simulink model "Sample594"  (R2021b)
settings: Solver=VariableStepAuto  StartTime=0.0  StopTime=10.0  RelTol=1e-3
undefined symbols (not defined in the file): DiscIntNeverNeededParam, magnitude, Newton, Raphson
libraries: simulink x402, pid_lib x98
(part 2 of 14)

== system Sample594/cfblk7/cfblk9 ==
  cfblk1 : Inport
  cfblk10 : Delay  SampleTime=1
  cfblk11 : Delay  SampleTime=1
  cfblk3 : simulink/Discrete/Difference  ICPrevInput=0.0  OutMin=[]  OutMax=[]  OutDataTypeStr=Inherit: Inherit via back propagation  OutDataType=fixdt(1, 16)  OutScaling=2^-10  DoSatur=off
  cfblk4 : simulink/Math Operations/Slider Gain  gain=1  low=0  high=2
  cfblk5 : Sum  Inputs=+
  cfblk6 : Subsystem
  cfblk7 : Subsystem
  cfblk8 : Subsystem
  cfblk9 : Delay  SampleTime=1
  cfblk2 : Outport
  wires:
  cfblk3/1 -> cfblk5/1
  cfblk1/1 -> cfblk2/1, cfblk6/2(cfblk15)
  cfblk8/1(cfblk2) -> cfblk9/1, cfblk10/1
  cfblk7/1(cfblk2) -> cfblk8/1(cfblk1)
  cfblk5/1 -> cfblk7/1(cfblk1), cfblk11/1
  cfblk4/1 -> cfblk7/2(cfblk7), cfblk7/3(cfblk8), cfblk7/4(cfblk9), cfblk3/1
  cfblk6/1(cfblk2) -> cfblk4/1
  cfblk9/1 -> cfblk6/1(cfblk1)
  cfblk10/1 -> cfblk6/3(cfblk16)
  cfblk11/1 -> cfblk6/4(cfblk17)

== system Sample594/cfblk8/cfblk10 ==
  cfblk1 : Inport
  cfblk9 : Inport  Port=2
  cfblk3 : Delay  DelayLengthSource=Input port  SampleTime=1
      settings: InputPortMap=u0,p1
  cfblk4 : Polyval  Coefs=[ +2.081618890e-019, -1.441693666e-014, +4.719686976e-010, -8.536869453e-006, +1.621573104e-001, -8.087801117e+001 ]
  cfblk5 : Assignment  DiagnosticForDimensions=Warning  IndexOptions=Index vector (dialog)  Indices=1  OutputSizes=1
  cfblk6 : Polyval  Coefs=[ +2.081618890e-019, -1.441693666e-014, +4.719686976e-010, -8.536869453e-006, +1.621573104e-001, -8.087801117e+001 ]
  cfblk7 : Constant  Value=[-685362202.844304]  SampleTime=1
  cfblk8 : Subsystem
  cfblk2 : Outport
  cfblk10 : Outport  Port=2
  cfblk11 : Outport  Port=3
  wires:
  cfblk5/1 -> cfblk6/1
  cfblk6/1 -> cfblk4/1
  cfblk8/1(cfblk2) -> cfblk2/1
  cfblk8/2(cfblk15) -> cfblk11/1
  cfblk1/1 -> cfblk5/1, cfblk8/4(cfblk14)
  cfblk9/1 -> cfblk5/2, cfblk8/3(cfblk13)
  cfblk4/1 -> cfblk10/1
  cfblk7/1 -> cfblk3/1, cfblk3/2
  cfblk3/1 -> cfblk8/1(cfblk1), cfblk8/2(cfblk12)

== system Sample594/cfblk8/cfblk11 ==
  cfblk1 : Inport
  cfblk13 : Inport  Port=2
  cfblk14 : Inport  Port=3
  cfblk10 : Subsystem
  cfblk11 : Subsystem
  cfblk12 : Subsystem
  cfblk15 : Delay  SampleTime=1
  cfblk16 : Delay  SampleTime=1
  cfblk3 : simulink/Discrete/Tapped Delay  vinit=0.0  samptime=-1  NumDelays=1  DelayOrder=Oldest  includeCurrent=off
  cfblk4 : DiscreteFilter  SampleTime=1
  cfblk5 : Abs
  cfblk6 : Reshape
  cfblk7 : simulink/Math Operations/Slider Gain  gain=1  low=0  high=2
  cfblk8 : PermuteDimensions
  cfblk9 : Subsystem
  cfblk2 : Outport
  wires:
  cfblk12/1(cfblk2) -> cfblk8/1
  cfblk13/1 -> cfblk6/1
  cfblk8/1 -> cfblk7/1
  cfblk7/1 -> cfblk4/1
  cfblk1/1 -> cfblk12/1(cfblk1)
  cfblk6/1 -> cfblk10/1(cfblk1)
  cfblk10/1(cfblk2) -> cfblk5/1
  cfblk4/1 -> cfblk9/1(cfblk1)
  cfblk14/1 -> cfblk11/1(cfblk1)
  cfblk9/2(cfblk7) -> cfblk11/2(cfblk13)
  cfblk12/2(cfblk16) -> cfblk9/2(cfblk6)
  cfblk10/2(cfblk12) -> cfblk11/3(cfblk14)
  cfblk9/3(cfblk8) -> cfblk2/1
  cfblk3/1 -> cfblk10/2(cfblk11)
  cfblk9/1(cfblk2) -> cfblk15/1
  cfblk15/1 -> cfblk12/2(cfblk15)
  cfblk5/1 -> cfblk16/1
  cfblk16/1 -> cfblk3/1

== system Sample594/cfblk8/cfblk12 ==
  cfblk1 : Inport
  cfblk13 : Inport  Port=2
  cfblk10 : Subsystem
  cfblk11 : Subsystem
  cfblk12 : If  IfExpression=u1 >= 0  SampleTime=1
  cfblk15 : Subsystem  TreatAsAtomicUnit=on
  cfblk16 : Subsystem  TreatAsAtomicUnit=on
  cfblk17 : Delay  SampleTime=1
  cfblk18 : Delay  SampleTime=1
  cfblk3 : Delay  ShowEnablePort=on  SampleTime=1
      settings: InputPortMap=u0,e6
  cfblk4 : pid_lib/PID Controller  Controller=PID  Form=Parallel  TimeDomain=Discrete-time  UseExternalTs=off  SampleTime=1  IntegratorMethod=Forward Euler  FilterMethod=Forward Euler  ControllerParametersSource=internal  P=1  I=1  D=0  UseFilter=on  N=100  TunerSelectOption=Transfer Function Based (PID Tuner App)  InitialConditionSource=internal  InitialConditionForIntegrator=0  InitialConditionForFilter=0  DifferentiatorICPrevScaledInput=0  ExternalReset=none  TrackingMode=off  Kt=1  LimitOutput=off  SatLimitsSource=internal  UpperSaturationLimit=inf  LowerSaturationLimit=-inf  LinearizeAsGain=off  AntiWindupMode=none  Kb=1  POutMin=[]  POutMax=[]  IOutMin=[]  IOutMax=[]  DOutMin=[]  DOutMax=[]  NOutMin=[]  NOutMax=[]  SumOutMin=[]  SumOutMax=[]  SaturationOutMin=[]  SaturationOutMax=[]  PParamMin=[]  PParamMax=[]  IParamMin=[]  IParamMax=[]  DParamMin=[]  DParamMax=[]  NParamMin=[]  NParamMax=[]  KbParamMin=[]  KbParamMax=[]  KtParamMin=[]  KtParamMax=[]  KbOutMin=[]  KbOutMax=[]  KtOutMin=[]  KtOutMax=[]  IntegratorOutMin=[]  IntegratorOutMax=[]  FilterOutMin=[]  FilterOutMax=[]  SumI1OutMin=[]  SumI1OutMax=[]  SumI2OutMin=[]  SumI2OutMax=[]  SumI3OutMin=[]  SumI3OutMax=[]  SumI4OutMin=[]  SumI4OutMax=[]  SumDOutMin=[]  SumDOutMax=[]  DifferentiatorOutMin=[]  DifferentiatorOutMax=[]  FilterDiffOutCoefMin=[]  FilterDiffOutCoefMax=[]  ReciprocalOutMin=[]  ReciprocalOutMax=[]  SumDenOutMin=[]  SumDenOutMax=[]  SumNumOutMin=[]  SumNumOutMax=[]  DivideOutMin=[]  DivideOutMax=[]  UdiffTsProdOutMin=[]  UdiffTsProdOutMax=[]  NTsProdOutMin=[]  NTsProdOutMax=[]  UintegralTsProdOutMin=[]  UintegralTsProdOutMax=[]  UngainTsProdOutMin=[]  UngainTsProdOutMax=[]  IntegratorContinuousStateAttributes=''  IntegratorStateMustResolveToSignalObject=off  IntegratorRTWStateStorageClass=Auto  FilterContinuousStateAttributes=''  FilterStateMustResolveToSignalObject=off  FilterRTWStateStorageClass=Auto  ParallelPVariant=InternalParameters  IdealPVariant=Disabled  IVariant=InternalParameters  DVariant=InternalParameters  IntegratorVariant=Discrete  SatVariant=Disabled  AWVariant=Passthrough  PCopyVariant=Disabled  TRVariant=Disabled  FdbkBlocksVariant=Forward  IdealPFdbkVariant=Disabled  SatFdbkVariant=Disabled  DerivativeFilterVariant=ForwardEulerFilter  NVariant=InternalParameters  NCopyVariant=Disabled  FilterICVariant=InternalICsFilter  IntegratorICVariant=InternalICs  ExternalResetVariant=Disabled  TRSumVariant=Passthrough  SumFdbkVariant=Disabled  SumVariant=Sum_PID  TsampFilterVariant=InternalTs  TsampNgainVariant=Passthrough  TsampIntegralVariant=Passthrough  ExternalSaturationOutDataTypeStr=Inherit: Same as second input
  cfblk5 : Rounding
  cfblk6 : PermuteDimensions
  cfblk7 : Polyval  Coefs=[ +2.081618890e-019, -1.441693666e-014, +4.719686976e-010, -8.536869453e-006, +1.621573104e-001, -8.087801117e+001 ]
  cfblk8 : Constant  Value=[-411590028.519686]  SampleTime=1
  cfblk9 : Subsystem
  cfblk2 : Outport
  cfblk14 : Outport  Port=2
  wires:
  cfblk11/1(cfblk2) -> cfblk4/1
  cfblk8/1 -> cfblk11/1(cfblk1)
  cfblk13/1 -> cfblk6/1
  cfblk4/1 -> cfblk3/1
  cfblk6/1 -> cfblk10/1(cfblk1)
  cfblk10/1(cfblk2) -> cfblk9/1(cfblk1)
  cfblk7/1 -> cfblk16/2(cfblk16)
  cfblk9/1(cfblk2) -> cfblk2/1
  cfblk5/1 -> cfblk7/1
  cfblk16/1(cfblk2) -> cfblk15/1(cfblk1)
  cfblk1/1 -> cfblk5/1, cfblk3/2
  cfblk3/1 -> cfblk14/1
  cfblk9/2(cfblk11) -> cfblk15/2(cfblk16)
  cfblk9/3(cfblk12) -> cfblk12/1
  cfblk12/1 -> cfblk15/Action
  cfblk12/2 -> cfblk16/Action
  cfblk15/1(cfblk2) -> cfblk17/1
  cfblk17/1 -> cfblk16/1(cfblk1)
  cfblk15/2(cfblk17) -> cfblk18/1
  cfblk18/1 -> cfblk16/3(cfblk17)

== system Sample594/cfblk8/cfblk13 ==
  cfblk1 : Inport
  cfblk6 : Inport  Port=2
  cfblk7 : Inport  Port=3
  cfblk3 : Gain  Gain=[833103995.126030]
  cfblk4 : Constant  Value=[-958629368.502449]  SampleTime=1
  cfblk5 : Subsystem
  cfblk2 : Outport
  wires:
  cfblk6/1 -> cfblk3/1
  cfblk5/1(cfblk2) -> cfblk2/1
  cfblk1/1 -> cfblk5/1(cfblk1)
  cfblk7/1 -> cfblk5/2(cfblk8)

== system Sample594/cfblk8/cfblk9 ==
  cfblk1 : Inport
  cfblk11 : Inport  Port=2
  cfblk12 : Inport  Port=3
  cfblk10 : Subsystem
  cfblk13 : Delay  SampleTime=1
  cfblk3 : simulink/Math Operations/MinMax Running Resettable  Function=min  vinit=0.0
  cfblk4 : Rounding
  cfblk5 : UnaryMinus
  cfblk6 : Subsystem
  cfblk7 : Subsystem
  cfblk8 : Subsystem
  cfblk9 : Subsystem
  cfblk2 : Outport
  wires:
  cfblk1/1 -> cfblk4/1, cfblk6/5(cfblk11)
  cfblk10/1(cfblk2) -> cfblk7/1(cfblk1)
  cfblk8/1(cfblk2) -> cfblk10/1(cfblk1)
  cfblk8/2(cfblk8) -> cfblk5/1
  cfblk5/1 -> cfblk9/1(cfblk1)
  cfblk12/1 -> cfblk3/1, cfblk6/3(cfblk9)
  cfblk7/1(cfblk2) -> cfblk6/1(cfblk1)
  cfblk6/1(cfblk2) -> cfblk2/1, cfblk13/1
  cfblk3/1 -> cfblk8/1(cfblk1)
  cfblk4/1 -> cfblk8/2(cfblk7), cfblk6/4(cfblk10)
  cfblk9/1(cfblk2) -> cfblk6/2(cfblk8), cfblk7/3(cfblk10)
  cfblk11/1 -> cfblk3/2
  cfblk13/1 -> cfblk7/2(cfblk9)

== system Sample594/cfblk9/cfblk14 ==
  cfblk1 : Inport
  cfblk10 : Inport  Port=2
  cfblk11 : Inport  Port=3
  cfblk12 : Inport  Port=4
  cfblk13 : Inport  Port=5
  cfblk17 : Delay  SampleTime=1
  cfblk3 : DiscreteZeroPole  Poles=[0 0.5]  Gain=1
  cfblk4 : DiscreteZeroPole  Poles=[0 0.5]  Gain=1
  cfblk5 : Sum  Inputs=+-
  cfblk6 : DotProduct  InputSameDT=on  OutDataTypeStr=Inherit: Inherit via internal rule
  cfblk7 : Constant  Value=[-386291814.551287]  SampleTime=1
  cfblk8 : Subsystem
  cfblk9 : Subsystem
  cfblk2 : Outport
  cfblk14 : Outport  Port=2
  cfblk15 : Outport  Port=3
  cfblk16 : Outport  Port=4
  wires:
  cfblk10/1 -> cfblk8/1(cfblk1)
  cfblk1/1 -> cfblk15/1, cfblk8/3(cfblk8)
  cfblk5/1 -> cfblk14/1
  cfblk8/1(cfblk2) -> cfblk9/1(cfblk1)
  cfblk12/1 -> cfblk5/1
  cfblk6/1 -> cfblk16/1
  cfblk11/1 -> cfblk4/1
  cfblk9/1(cfblk2) -> cfblk3/1
  cfblk7/1 -> cfblk5/2
  cfblk13/1 -> cfblk6/1
  cfblk4/1 -> cfblk6/2, cfblk2/1, cfblk9/2(cfblk12)
  cfblk3/1 -> cfblk17/1
  cfblk17/1 -> cfblk8/2(cfblk7)

== system Sample594/cfblk11/cfblk10/cfblk10 ==
  cfblk1 : Inport
  cfblk10 : Subsystem
  cfblk{11..14} (4 alike) : Delay
  cfblk3 : Abs
  cfblk4 : Sum  Inputs=--
  cfblk5 : simulink/Math Operations/Slider Gain  gain=1  low=0  high=2
  cfblk6 : Signum
  cfblk7 : Subsystem
  cfblk8 : Subsystem
  cfblk9 : Subsystem
  cfblk2 : Outport
  wires:
  cfblk3/1 -> cfblk7/3(cfblk15), cfblk14/1
  cfblk4/1 -> cfblk10/1(cfblk1), cfblk7/4(cfblk16)
  cfblk5/1 -> cfblk4/2
  cfblk8/1(cfblk2) -> cfblk2/1
  cfblk8/2(cfblk10) -> cfblk6/1
  cfblk10/1(cfblk2) -> cfblk3/1, cfblk13/1
  cfblk1/1 -> cfblk8/3(cfblk9), cfblk7/2(cfblk14)
  cfblk8/3(cfblk11) -> cfblk9/2(cfblk9)
  cfblk9/1(cfblk2) -> cfblk7/1(cfblk1), cfblk5/1, cfblk7/5(cfblk17)
  cfblk6/1 -> cfblk11/1
  cfblk11/1 -> cfblk8/1(cfblk1)
  cfblk7/1(cfblk2) -> cfblk12/1
  cfblk12/1 -> cfblk8/2(cfblk8)
  cfblk13/1 -> cfblk9/1(cfblk1)
  cfblk14/1 -> cfblk4/1

== system Sample594/cfblk11/cfblk10/cfblk11 ==
  cfblk1 : Inport
  cfblk10 : Inport  Port=2
  cfblk11 : Delay
  cfblk12 : Delay
  cfblk13 : Delay
  cfblk3 : DiscreteIntegrator  SampleTime=-1  ICPrevOutput=DiscIntNeverNeededParam  ICPrevScaledInput=DiscIntNeverNeededParam
  cfblk4 : simulink/Math Operations/Slider Gain  gain=1  low=0  high=2
  cfblk5 : Abs
  cfblk6 : Sqrt  SaturateOnIntegerOverflow=on
  cfblk7 : Subsystem
  cfblk8 : Subsystem
  cfblk9 : Subsystem
  cfblk2 : Outport
  wires:
  cfblk8/1(cfblk2) -> cfblk6/1
  cfblk1/1 -> cfblk5/1
  cfblk7/1(cfblk2) -> cfblk4/1
  cfblk9/1(cfblk2) -> cfblk3/1
  cfblk6/1 -> cfblk7/2(cfblk14), cfblk9/3(cfblk14)
  cfblk10/1 -> cfblk8/2(cfblk13)
  cfblk8/2(cfblk15) -> cfblk7/3(cfblk15)
  cfblk8/3(cfblk16) -> cfblk2/1
  cfblk5/1 -> cfblk9/2(cfblk13), cfblk8/3(cfblk14)
  cfblk3/1 -> cfblk11/1
  cfblk11/1 -> cfblk9/1(cfblk1)
  cfblk4/1 -> cfblk12/1
  cfblk12/1 -> cfblk7/1(cfblk1)
  cfblk7/2(cfblk16) -> cfblk13/1
  cfblk13/1 -> cfblk8/1(cfblk1)

== system Sample594/cfblk11/cfblk10/cfblk12 ==
  cfblk1 : Inport
  cfblk10 : Inport  Port=2
  cfblk11 : Inport  Port=3
  cfblk3 : DiscreteTransferFcn
  cfblk4 : Sqrt  Operator=rSqrt  AlgorithmType=Newton-Raphson  SaturateOnIntegerOverflow=on
  cfblk5 : simulink/Math Operations/MinMax Running Resettable  Function=min  vinit=0.0
  cfblk6 : Sum  Inputs=--
  cfblk7 : Sin  TimeSource=Use external signal  SampleTime=0
  cfblk8 : Sqrt  Operator=rSqrt  AlgorithmType=Newton-Raphson  SaturateOnIntegerOverflow=on
  cfblk9 : Subsystem
  cfblk2 : Outport
  wires:
  cfblk11/1 -> cfblk8/1, cfblk9/6(cfblk14)
  cfblk8/1 -> cfblk3/1, cfblk9/3(cfblk11), cfblk9/5(cfblk13), cfblk9/7(cfblk15)
  cfblk7/1 -> cfblk2/1, cfblk9/1(cfblk1)
  cfblk4/1 -> cfblk6/1
  cfblk1/1 -> cfblk6/2
  cfblk3/1 -> cfblk4/1, cfblk9/4(cfblk12)
  cfblk5/1 -> cfblk7/1
  cfblk6/1 -> cfblk5/1
  cfblk10/1 -> cfblk5/2, cfblk9/2(cfblk10)

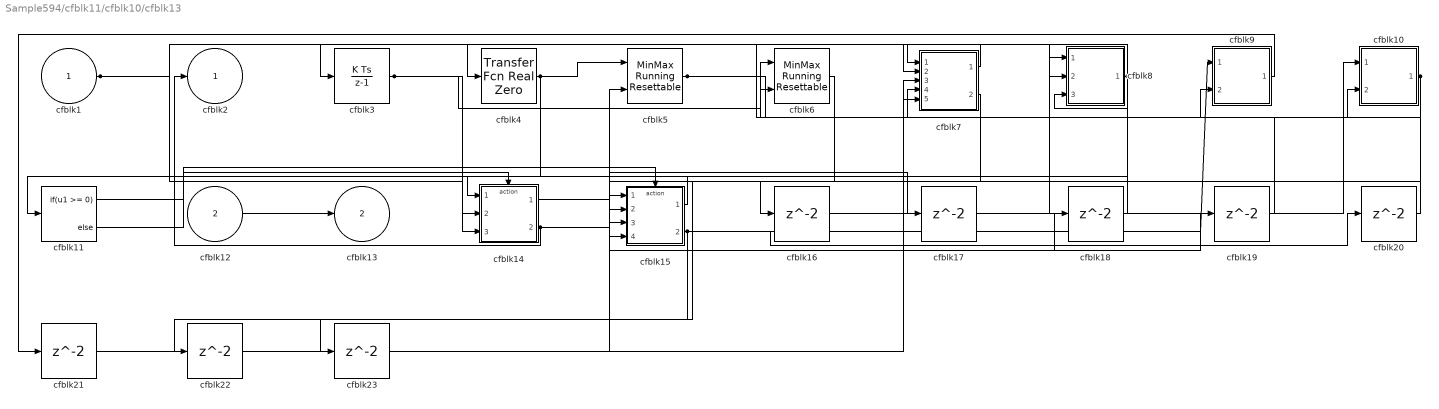
== system Sample594/cfblk11/cfblk10/cfblk13 ==
  cfblk1 : Inport
  cfblk12 : Inport  Port=2
  cfblk10 : Subsystem
  cfblk11 : If  IfExpression=u1 >= 0  SampleTime=1
  cfblk14 : Subsystem  TreatAsAtomicUnit=on
  cfblk15 : Subsystem  TreatAsAtomicUnit=on
  cfblk{16..23} (8 alike) : Delay
  cfblk3 : DiscreteIntegrator  SampleTime=-1  ICPrevOutput=DiscIntNeverNeededParam  ICPrevScaledInput=DiscIntNeverNeededParam
  cfblk4 : simulink/Discrete/Transfer Fcn Real Zero  ZeroZ=0.75  ICPrevInput=0.0  DoSatur=off
      settings: SourceProductBaseCode=SL
  cfblk5 : simulink/Math Operations/MinMax Running Resettable  Function=min  vinit=0.0
  cfblk6 : simulink/Math Operations/MinMax Running Resettable  Function=min  vinit=0.0
  cfblk7 : Subsystem
  cfblk8 : Subsystem
  cfblk9 : Subsystem
  cfblk2 : Outport
  cfblk13 : Outport  Port=2
  wires:
  cfblk8/1(cfblk2) -> cfblk4/1, cfblk11/1, cfblk7/2(cfblk13), cfblk15/3(cfblk13)
  cfblk14/2(cfblk17) -> cfblk2/1, cfblk18/1, cfblk19/1
  cfblk3/1 -> cfblk6/1, cfblk15/4(cfblk14)
  cfblk10/1(cfblk2) -> cfblk7/4(cfblk15), cfblk16/1
  cfblk15/1(cfblk2) -> cfblk14/1(cfblk1)
  cfblk4/1 -> cfblk5/1, cfblk14/3(cfblk16)
  cfblk1/1 -> cfblk8/2(cfblk9), cfblk14/2(cfblk15)
  cfblk7/1(cfblk2) -> cfblk3/1
  cfblk6/1 -> cfblk15/2(cfblk12)
  cfblk12/1 -> cfblk13/1
  cfblk5/1 -> cfblk10/2(cfblk7), cfblk7/1(cfblk1), cfblk9/2(cfblk11)
  cfblk15/2(cfblk15) -> cfblk9/1(cfblk1), cfblk20/1, cfblk22/1
  cfblk11/1 -> cfblk14/Action
  cfblk11/2 -> cfblk15/Action
  cfblk16/1 -> cfblk8/1(cfblk1)
  cfblk14/1(cfblk2) -> cfblk17/1
  cfblk17/1 -> cfblk10/1(cfblk1)
  cfblk18/1 -> cfblk8/3(cfblk10)
  cfblk19/1 -> cfblk7/3(cfblk14)
  cfblk20/1 -> cfblk6/2
  cfblk9/1(cfblk2) -> cfblk21/1
  cfblk21/1 -> cfblk15/1(cfblk1)
  cfblk22/1 -> cfblk7/5(cfblk16)
  cfblk7/2(cfblk17) -> cfblk23/1
  cfblk23/1 -> cfblk5/2

== system Sample594/cfblk11/cfblk11/cfblk10 ==
  cfblk1 : Inport
  cfblk9 : Inport  Port=2
  cfblk10 : Subsystem  TreatAsAtomicUnit=on
  cfblk11 : Subsystem  TreatAsAtomicUnit=on
  cfblk{12..15} (4 alike) : Delay
  cfblk3 : Signum
  cfblk4 : Signum
  cfblk5 : Reshape
  cfblk6 : Math  Operator=pow  SaturateOnIntegerOverflow=on
  cfblk7 : Subsystem
  cfblk8 : If  IfExpression=u1 >= 0  SampleTime=1
  cfblk2 : Outport
  wires:
  cfblk4/1 -> cfblk7/1(cfblk1)
  cfblk11/2(cfblk13) -> cfblk5/1
  cfblk1/1 -> cfblk3/1
  cfblk5/1 -> cfblk7/2(cfblk9)
  cfblk10/1(cfblk2) -> cfblk6/1
  cfblk10/2(cfblk7) -> cfblk2/1
  cfblk9/1 -> cfblk4/1
  cfblk7/1(cfblk2) -> cfblk6/2
  cfblk3/1 -> cfblk11/1(cfblk1)
  cfblk8/1 -> cfblk10/Action
  cfblk8/2 -> cfblk11/Action
  cfblk6/1 -> cfblk12/1
  cfblk12/1 -> cfblk10/1(cfblk1)
  cfblk11/1(cfblk2) -> cfblk13/1
  cfblk13/1 -> cfblk8/1
  cfblk7/2(cfblk10) -> cfblk14/1
  cfblk14/1 -> cfblk11/2(cfblk11)
  cfblk7/3(cfblk11) -> cfblk15/1
  cfblk15/1 -> cfblk11/3(cfblk12)

== system Sample594/cfblk11/cfblk11/cfblk11 ==
  cfblk1 : Inport
  cfblk10 : Inport  Port=2
  cfblk11 : Inport  Port=3
  cfblk12 : Inport  Port=4
  cfblk3 : DiscreteZeroPole  Poles=[0 0.5]  Gain=1  SampleTime=-1
  cfblk4 : Delay  DelayLengthSource=Input port
      settings: InputPortMap=u0,p1
  cfblk5 : Reshape
  cfblk6 : Constant  Value=[-771785140.831917]  SampleTime=1
  cfblk7 : Subsystem
  cfblk8 : Subsystem
  cfblk9 : Subsystem
  cfblk2 : Outport
  cfblk13 : Outport  Port=2
  wires:
  cfblk1/1 -> cfblk5/1, cfblk7/4(cfblk16)
  cfblk5/1 -> cfblk9/1(cfblk1), cfblk7/1(cfblk1)
  cfblk3/1 -> cfblk4/1
  cfblk4/1 -> cfblk13/1
  cfblk10/1 -> cfblk8/1(cfblk1)
  cfblk8/1(cfblk2) -> cfblk4/2
  cfblk7/1(cfblk2) -> cfblk3/1
  cfblk12/1 -> cfblk9/2(cfblk11)
  cfblk6/1 -> cfblk9/3(cfblk12), cfblk7/3(cfblk15)
  cfblk11/1 -> cfblk2/1
  cfblk9/1(cfblk2) -> cfblk8/2(cfblk13)
  cfblk9/2(cfblk13) -> cfblk8/3(cfblk14), cfblk7/2(cfblk14)

== system Sample594/cfblk11/cfblk11/cfblk12 ==
  cfblk1 : Inport
  cfblk12 : Delay
  cfblk13 : Delay
  cfblk14 : Delay
  cfblk3 : Polyval  Coefs=[ +2.081618890e-019, -1.441693666e-014, +4.719686976e-010, -8.536869453e-006, +1.621573104e-001, -8.087801117e+001 ]
  cfblk4 : Signum
  cfblk5 : simulink/Math Operations/Slider Gain  gain=1  low=0  high=2
  cfblk6 : Subsystem
  cfblk7 : Subsystem
  cfblk8 : Subsystem
  cfblk2 : Outport
  cfblk9 : Outport  Port=2
  cfblk10 : Outport  Port=3
  cfblk11 : Outport  Port=4
  wires:
  cfblk1/1 -> cfblk4/1, cfblk5/1
  cfblk8/1(cfblk2) -> cfblk9/1
  cfblk5/1 -> cfblk6/1(cfblk1), cfblk7/2(cfblk9), cfblk6/4(cfblk13)
  cfblk3/1 -> cfblk8/3(cfblk12), cfblk12/1, cfblk13/1
  cfblk4/1 -> cfblk11/1, cfblk8/2(cfblk11), cfblk6/3(cfblk12), cfblk8/4(cfblk13), cfblk8/5(cfblk14), cfblk8/6(cfblk15)
  cfblk7/1(cfblk2) -> cfblk3/1
  cfblk6/1(cfblk2) -> cfblk7/1(cfblk1)
  cfblk7/2(cfblk11) -> cfblk10/1
  cfblk7/3(cfblk12) -> cfblk8/1(cfblk1), cfblk2/1, cfblk14/1
  cfblk12/1 -> cfblk6/2(cfblk11)
  cfblk13/1 -> cfblk7/3(cfblk10)
  cfblk14/1 -> cfblk6/5(cfblk14)

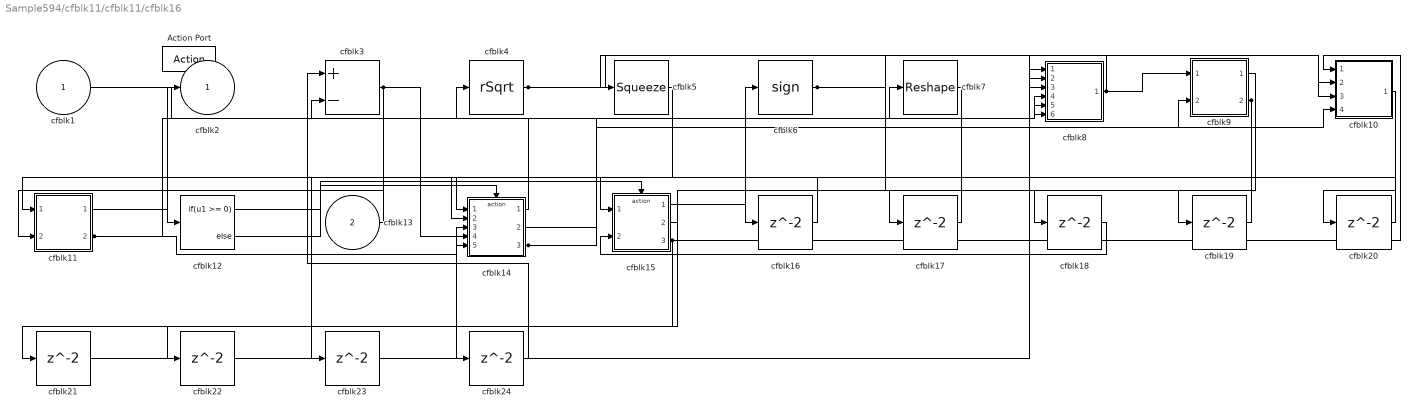
== system Sample594/cfblk11/cfblk11/cfblk16 ==
  cfblk1 : Inport
  cfblk13 : Inport  Port=2
  Action Port : ActionPort  ActionPortLabel=if(u1 >= 0)
  cfblk10 : Subsystem
  cfblk11 : Subsystem
  cfblk12 : If  IfExpression=u1 >= 0  SampleTime=1
  cfblk14 : Subsystem  TreatAsAtomicUnit=on
  cfblk15 : Subsystem  TreatAsAtomicUnit=on
  cfblk{16..24} (9 alike) : Delay
  cfblk3 : Sum  Inputs=+-
  cfblk4 : Sqrt  Operator=rSqrt  AlgorithmType=Newton-Raphson  SaturateOnIntegerOverflow=on
  cfblk5 : Squeeze
  cfblk6 : Signum
  cfblk7 : Reshape
  cfblk8 : Subsystem
  cfblk9 : Subsystem
  cfblk2 : Outport
  wires:
  cfblk13/1 -> cfblk12/1
  cfblk1/1 -> cfblk3/2
  cfblk8/1(cfblk2) -> cfblk9/1(cfblk1), cfblk5/1
  cfblk15/1(cfblk2) -> cfblk6/1
  cfblk9/2(cfblk8) -> cfblk17/1, cfblk18/1
  cfblk6/1 -> cfblk10/3(cfblk12), cfblk19/1
  cfblk15/3(cfblk16) -> cfblk10/1(cfblk1), cfblk22/1
  cfblk11/1(cfblk2) -> cfblk2/1
  cfblk14/1(cfblk2) -> cfblk4/1
  cfblk3/1 -> cfblk11/2(cfblk8), cfblk14/4(cfblk8)
  cfblk14/2(cfblk10) -> cfblk7/1
  cfblk14/3(cfblk11) -> cfblk9/2(cfblk7), cfblk10/4(cfblk13), cfblk8/6(cfblk15)
  cfblk4/1 -> cfblk8/3(cfblk12), cfblk10/2(cfblk11)
  cfblk11/2(cfblk9) -> cfblk14/3(cfblk7), cfblk8/4(cfblk13), cfblk8/5(cfblk14)
  cfblk12/1 -> cfblk14/Action
  cfblk12/2 -> cfblk15/Action
  cfblk9/1(cfblk2) -> cfblk16/1
  cfblk16/1 -> cfblk14/2(cfblk6)
  cfblk17/1 -> cfblk11/1(cfblk1)
  cfblk18/1 -> cfblk15/2(cfblk14)
  cfblk19/1 -> cfblk15/1(cfblk1)
  cfblk10/1(cfblk2) -> cfblk20/1
  cfblk20/1 -> cfblk14/1(cfblk1)
  cfblk15/2(cfblk15) -> cfblk21/1
  cfblk21/1 -> cfblk8/2(cfblk11)
  cfblk22/1 -> cfblk14/5(cfblk9)
  cfblk5/1 -> cfblk23/1
  cfblk23/1 -> cfblk8/1(cfblk1)
  cfblk7/1 -> cfblk24/1
  cfblk24/1 -> cfblk3/1

== system Sample594/cfblk11/cfblk11/cfblk17 ==
  cfblk1 : Inport
  Action Port : ActionPort  ActionPortLabel=else
  cfblk3 : Sum  Inputs=|++
  cfblk4 : Squeeze
  cfblk5 : Constant  Value=[614173077.756830]  SampleTime=1
  cfblk6 : Subsystem
  cfblk7 : Subsystem
  cfblk2 : Outport
  wires:
  cfblk1/1 -> cfblk6/1(cfblk1)
  cfblk6/1(cfblk2) -> cfblk3/1
  cfblk5/1 -> cfblk2/1
  cfblk3/1 -> cfblk7/1(cfblk1)
  cfblk4/1 -> cfblk3/2
  cfblk6/2(cfblk6) -> cfblk7/2(cfblk15)
  cfblk6/3(cfblk7) -> cfblk4/1
  cfblk6/4(cfblk8) -> cfblk7/3(cfblk16)

== system Sample594/cfblk11/cfblk12/cfblk12 ==
  cfblk1 : Inport
  cfblk12 : Inport  Port=2
  cfblk13 : Inport  Port=3
  cfblk14 : Inport  Port=4
  cfblk10 : Subsystem
  cfblk11 : Subsystem
  cfblk15 : Delay
  cfblk16 : Delay
  cfblk3 : Delay
  cfblk4 : DotProduct  InputSameDT=on  OutDataTypeStr=Inherit: Inherit via internal rule
  cfblk5 : Abs
  cfblk6 : PermuteDimensions
  cfblk7 : DotProduct  InputSameDT=on  OutDataTypeStr=Inherit: Inherit via internal rule
  cfblk8 : Subsystem
  cfblk9 : Subsystem
  cfblk2 : Outport
  wires:
  cfblk3/1 -> cfblk9/1(cfblk1)
  cfblk7/1 -> cfblk9/2(cfblk13)
  cfblk8/1(cfblk2) -> cfblk4/1
  cfblk8/2(cfblk14) -> cfblk3/1
  cfblk8/3(cfblk15) -> cfblk11/1(cfblk1)
  cfblk9/1(cfblk2) -> cfblk2/1
  cfblk1/1 -> cfblk4/2
  cfblk9/2(cfblk16) -> cfblk11/2(cfblk12)
  cfblk14/1 -> cfblk9/3(cfblk14), cfblk11/4(cfblk14)
  cfblk6/1 -> cfblk11/3(cfblk13)
  cfblk12/1 -> cfblk10/1(cfblk1)
  cfblk13/1 -> cfblk6/1
  cfblk10/2(cfblk7) -> cfblk8/1(cfblk1), cfblk9/4(cfblk15)
  cfblk5/1 -> cfblk10/2(cfblk6)
  cfblk4/1 -> cfblk7/2
  cfblk11/1(cfblk2) -> cfblk15/1
  cfblk15/1 -> cfblk7/1
  cfblk10/1(cfblk2) -> cfblk16/1
  cfblk16/1 -> cfblk5/1

== system Sample594/cfblk11/cfblk12/cfblk13 ==
  cfblk1 : Inport
  cfblk7 : Inport  Port=2
  cfblk8 : Inport  Port=3
  cfblk10 : Subsystem  TreatAsAtomicUnit=on
  cfblk{11..14} (4 alike) : Delay
  cfblk3 : ComplexToMagnitudeAngle
  cfblk4 : simulink/Math Operations/MinMax Running Resettable  Function=min  vinit=0.0
  cfblk5 : Subsystem
  cfblk6 : If  IfExpression=u1 >= 0  SampleTime=1
  cfblk9 : Subsystem  TreatAsAtomicUnit=on
  cfblk2 : Outport
  wires:
  cfblk7/1 -> cfblk9/1(cfblk1), cfblk10/3(cfblk8)
  cfblk3/1 -> cfblk10/2(cfblk7)
  cfblk3/2 -> cfblk2/1
  cfblk5/1(cfblk2) -> cfblk6/1
  cfblk1/1 -> cfblk5/2(cfblk13), cfblk3/1
  cfblk5/2(cfblk16) -> cfblk9/2(cfblk13)
  cfblk8/1 -> cfblk9/3(cfblk14)
  cfblk9/1(cfblk2) -> cfblk4/1
  cfblk9/3(cfblk16) -> cfblk4/2, cfblk14/1
  cfblk6/1 -> cfblk9/Action
  cfblk6/2 -> cfblk10/Action
  cfblk4/1 -> cfblk11/1
  cfblk11/1 -> cfblk10/1(cfblk1)
  cfblk10/1(cfblk2) -> cfblk12/1
  cfblk12/1 -> cfblk5/1(cfblk1)
  cfblk9/2(cfblk15) -> cfblk13/1
  cfblk13/1 -> cfblk5/3(cfblk14)
  cfblk14/1 -> cfblk5/4(cfblk15)

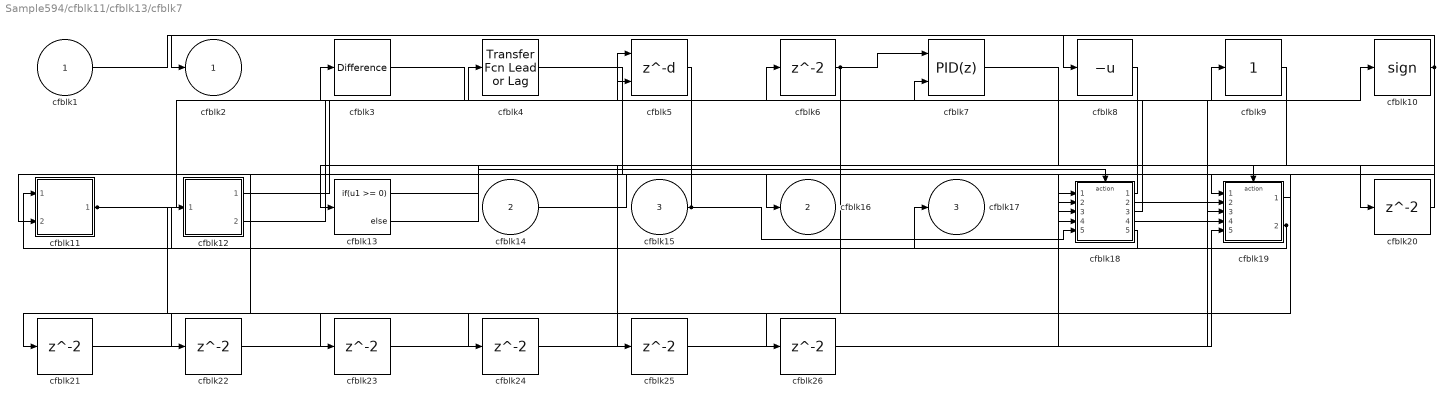
== system Sample594/cfblk11/cfblk13/cfblk7 ==
  cfblk1 : Inport
  cfblk14 : Inport  Port=2
  cfblk15 : Inport  Port=3
  cfblk10 : Signum
  cfblk11 : Subsystem
  cfblk12 : Subsystem
  cfblk13 : If  IfExpression=u1 >= 0  SampleTime=1
  cfblk18 : Subsystem  TreatAsAtomicUnit=on
  cfblk19 : Subsystem  TreatAsAtomicUnit=on
  cfblk{6,20..26} (8 alike) : Delay
  cfblk3 : simulink/Discrete/Difference  ICPrevInput=0.0  OutMin=[]  OutMax=[]  OutDataTypeStr=Inherit: Inherit via back propagation  OutDataType=fixdt(1, 16)  OutScaling=2^-10  DoSatur=off
  cfblk4 : simulink/Discrete/Transfer Fcn Lead or Lag  PoleZ=0.95  ZeroZ=0.75  ICPrevOutput=0.0  ICPrevInput=0.0  DoSatur=off
      settings: SourceProductBaseCode=SL
  cfblk5 : Delay  DelayLengthSource=Input port
      settings: InputPortMap=u0,p1
  cfblk7 : pid_lib/PID Controller (2DOF)  Controller=PID  Form=Parallel  TimeDomain=Discrete-time  UseExternalTs=off  SampleTime=-1  IntegratorMethod=Forward Euler  FilterMethod=Forward Euler  ControllerParametersSource=internal  P=1  I=1  D=0  UseFilter=on  N=100  b=1  c=1  TunerSelectOption=Transfer Function Based (PID Tuner App)  InitialConditionSource=internal  InitialConditionForIntegrator=0  InitialConditionForFilter=0  DifferentiatorICPrevScaledInput=0  ExternalReset=none  TrackingMode=off  Kt=1  LimitOutput=off  SatLimitsSource=internal  UpperSaturationLimit=inf  LowerSaturationLimit=-inf  LinearizeAsGain=off  AntiWindupMode=none  Kb=1  POutMin=[]  POutMax=[]  IOutMin=[]  IOutMax=[]  DOutMin=[]  DOutMax=[]  NOutMin=[]  NOutMax=[]  bOutMin=[]  bOutMax=[]  cOutMin=[]  cOutMax=[]  SumOutMin=[]  SumOutMax=[]  SaturationOutMin=[]  SaturationOutMax=[]  PParamMin=[]  PParamMax=[]  IParamMin=[]  IParamMax=[]  DParamMin=[]  DParamMax=[]  NParamMin=[]  NParamMax=[]  bParamMin=[]  bParamMax=[]  cParamMin=[]  cParamMax=[]  KbParamMin=[]  KbParamMax=[]  KtParamMin=[]  KtParamMax=[]  KbOutMin=[]  KbOutMax=[]  KtOutMin=[]  KtOutMax=[]  IntegratorOutMin=[]  IntegratorOutMax=[]  FilterOutMin=[]  FilterOutMax=[]  SumI1OutMin=[]  SumI1OutMax=[]  SumI2OutMin=[]  SumI2OutMax=[]  SumI3OutMin=[]  SumI3OutMax=[]  SumI4OutMin=[]  SumI4OutMax=[]  SumDOutMin=[]  SumDOutMax=[]  Sum1OutMin=[]  Sum1OutMax=[]  Sum2OutMin=[]  Sum2OutMax=[]  Sum3OutMin=[]  Sum3OutMax=[]  DifferentiatorOutMin=[]  DifferentiatorOutMax=[]  FilterDiffOutCoefMin=[]  FilterDiffOutCoefMax=[]  ReciprocalOutMin=[]  ReciprocalOutMax=[]  SumDenOutMin=[]  SumDenOutMax=[]  SumNumOutMin=[]  SumNumOutMax=[]  DivideOutMin=[]  DivideOutMax=[]  UdiffTsProdOutMin=[]  UdiffTsProdOutMax=[]  NTsProdOutMin=[]  NTsProdOutMax=[]  UintegralTsProdOutMin=[]  UintegralTsProdOutMax=[]  UngainTsProdOutMin=[]  UngainTsProdOutMax=[]  IntegratorContinuousStateAttributes=''  IntegratorStateMustResolveToSignalObject=off  IntegratorRTWStateStorageClass=Auto  FilterContinuousStateAttributes=''  FilterStateMustResolveToSignalObject=off  FilterRTWStateStorageClass=Auto  ParallelPVariant=InternalParameters  IdealPVariant=Disabled  IVariant=InternalParameters  DVariant=InternalParameters  bVariant=InternalParameters  cVariant=InternalParameters  IntegratorVariant=Discrete  SatVariant=Disabled  AWVariant=Passthrough  PCopyVariant=Disabled  TRVariant=Disabled  FdbkBlocksVariant=Forward  IdealPFdbkVariant=Disabled  SatFdbkVariant=Disabled  DerivativeFilterVariant=ForwardEulerFilter  NVariant=InternalParameters  NCopyVariant=Disabled  FilterICVariant=InternalICsFilter  IntegratorICVariant=InternalICs  ExternalResetVariant=Disabled  TRSumVariant=Passthrough  SumFdbkVariant=Disabled  SumVariant=Sum_PID  TsampFilterVariant=InternalTs  TsampNgainVariant=Passthrough  TsampIntegralVariant=Passthrough  ExternalSaturationOutDataTypeStr=Inherit: Same as second input
      settings: SourceProductBaseCode=SL
  cfblk8 : UnaryMinus
  cfblk9 : simulink/Math Operations/Slider Gain  gain=1  low=0  high=2
  cfblk2 : Outport
  cfblk16 : Outport  Port=2
  cfblk17 : Outport  Port=3
  wires:
  cfblk14/1 -> cfblk19/1(cfblk1)
  cfblk6/1 -> cfblk7/1, cfblk23/1
  cfblk12/1(cfblk2) -> cfblk4/1
  cfblk10/1 -> cfblk2/1, cfblk11/2(cfblk12), cfblk24/1
  cfblk4/1 -> cfblk16/1
  cfblk15/1 -> cfblk3/1, cfblk18/5(cfblk13)
  cfblk1/1 -> cfblk8/1
  cfblk18/1(cfblk2) -> cfblk6/1
  cfblk18/2(cfblk14) -> cfblk19/2(cfblk12)
  cfblk11/1(cfblk2) -> cfblk9/1, cfblk26/1
  cfblk12/2(cfblk9) -> cfblk5/1
  cfblk19/2(cfblk16) -> cfblk17/1, cfblk12/1(cfblk1)
  cfblk18/3(cfblk15) -> cfblk7/2
  cfblk8/1 -> cfblk18/3(cfblk11)
  cfblk18/4(cfblk16) -> cfblk10/1
  cfblk18/5(cfblk17) -> cfblk11/1(cfblk1)
  cfblk3/1 -> cfblk5/2
  cfblk13/1 -> cfblk18/Action
  cfblk13/2 -> cfblk19/Action
  cfblk7/1 -> cfblk20/1
  cfblk20/1 -> cfblk13/1
  cfblk19/1(cfblk2) -> cfblk21/1
  cfblk21/1 -> cfblk18/1(cfblk1)
  cfblk5/1 -> cfblk22/1
  cfblk22/1 -> cfblk18/4(cfblk12)
  cfblk23/1 -> cfblk19/5(cfblk15)
  cfblk24/1 -> cfblk19/3(cfblk13)
  cfblk9/1 -> cfblk25/1
  cfblk25/1 -> cfblk18/2(cfblk10)
  cfblk26/1 -> cfblk19/4(cfblk14)

== system Sample594/cfblk11/cfblk13/cfblk8 ==
  cfblk1 : Inport
  cfblk9 : Inport  Port=2
  cfblk10 : Delay
  cfblk3 : Math  Operator=mod  SaturateOnIntegerOverflow=on
  cfblk4 : Constant  Value=[314046642.390570]  SampleTime=1
  cfblk5 : Constant  Value=[-600688154.135266]  SampleTime=1
  cfblk6 : Subsystem
  cfblk7 : Subsystem
  cfblk8 : Subsystem
  cfblk2 : Outport
  wires:
  cfblk7/1(cfblk2) -> cfblk8/2(cfblk9)
  cfblk7/2(cfblk9) -> cfblk6/1(cfblk1)
  cfblk5/1 -> cfblk7/1(cfblk1)
  cfblk1/1 -> cfblk7/2(cfblk6)
  cfblk7/3(cfblk10) -> cfblk6/2(cfblk12)
  cfblk8/1(cfblk2) -> cfblk2/1
  cfblk9/1 -> cfblk7/3(cfblk7)
  cfblk4/1 -> cfblk7/4(cfblk8)
  cfblk7/4(cfblk11) -> cfblk3/1
  cfblk8/2(cfblk10) -> cfblk3/2
  cfblk3/1 -> cfblk10/1
  cfblk10/1 -> cfblk8/1(cfblk1)

== system Sample594/cfblk11/cfblk13/cfblk9 ==
  cfblk1 : Inport
  cfblk10 : Subsystem
  cfblk11 : Subsystem
  cfblk{13..17} (5 alike) : Delay
  cfblk3 : Delay  DelayLengthSource=Input port
      settings: InputPortMap=u0,p1
  cfblk4 : Gain  Gain=[-748566319.824225]
  cfblk5 : Sum
  cfblk6 : Rounding
  cfblk7 : Squeeze
  cfblk8 : Sum  Inputs=+-
  cfblk9 : Constant  Value=[-619601350.335139]  SampleTime=1
  cfblk2 : Outport
  cfblk12 : Outport  Port=2
  wires:
  cfblk7/1 -> cfblk3/1
  cfblk10/1(cfblk2) -> cfblk14/1, cfblk15/1, cfblk16/1
  cfblk4/1 -> cfblk7/1, cfblk11/3(cfblk10)
  cfblk5/1 -> cfblk11/1(cfblk1)
  cfblk11/2(cfblk14) -> cfblk6/1, cfblk12/1
  cfblk3/1 -> cfblk5/1, cfblk11/4(cfblk11)
  cfblk8/1 -> cfblk4/1, cfblk10/2(cfblk13), cfblk11/2(cfblk9)
  cfblk9/1 -> cfblk2/1
  cfblk1/1 -> cfblk8/2
  cfblk6/1 -> cfblk10/1(cfblk1), cfblk17/1
  cfblk11/1(cfblk2) -> cfblk13/1
  cfblk13/1 -> cfblk8/1
  cfblk14/1 -> cfblk3/2
  cfblk15/1 -> cfblk11/5(cfblk12)
  cfblk16/1 -> cfblk11/6(cfblk13)
  cfblk17/1 -> cfblk5/2

== system Sample594/cfblk11/cfblk14/cfblk10 ==
  cfblk1 : Inport
  cfblk15 : Inport  Port=2
  cfblk10 : Subsystem
  cfblk11 : Subsystem
  cfblk12 : Subsystem
  cfblk13 : Subsystem
  cfblk14 : If  IfExpression=u1 >= 0  SampleTime=1
  cfblk18 : Subsystem  TreatAsAtomicUnit=on
  cfblk19 : Subsystem  TreatAsAtomicUnit=on
  cfblk20 : Delay
  cfblk21 : Delay
  cfblk22 : Delay
  cfblk3 : DiscreteFilter
  cfblk4 : Math  Operator=transpose  SaturateOnIntegerOverflow=on
  cfblk5 : DotProduct  InputSameDT=on  OutDataTypeStr=Inherit: Inherit via internal rule
  cfblk6 : Signum
  cfblk7 : Constant  Value=[788475650.613690]  SampleTime=1
  cfblk8 : Constant  Value=[-793207360.881274]  SampleTime=1
  cfblk9 : Constant  Value=[402704456.160526]  SampleTime=1
  cfblk2 : Outport
  cfblk16 : Outport  Port=2
  cfblk17 : Outport  Port=3
  wires:
  cfblk13/1(cfblk2) -> cfblk11/1(cfblk1)
  cfblk11/1(cfblk2) -> cfblk5/1
  cfblk4/1 -> cfblk12/1(cfblk1)
  cfblk6/1 -> cfblk14/1
  cfblk3/1 -> cfblk5/2
  cfblk13/2(cfblk13) -> cfblk10/1(cfblk1)
  cfblk8/1 -> cfblk10/2(cfblk14)
  cfblk9/1 -> cfblk13/1(cfblk1)
  cfblk19/1(cfblk2) -> cfblk16/1
  cfblk10/1(cfblk2) -> cfblk17/1
  cfblk5/1 -> cfblk19/1(cfblk1)
  cfblk1/1 -> cfblk3/1
  cfblk7/1 -> cfblk6/1
  cfblk13/3(cfblk14) -> cfblk19/2(cfblk7)
  cfblk19/2(cfblk8) -> cfblk10/3(cfblk15)
  cfblk15/1 -> cfblk2/1
  cfblk11/2(cfblk7) -> cfblk18/2(cfblk11)
  cfblk14/1 -> cfblk18/Action
  cfblk14/2 -> cfblk19/Action
  cfblk10/2(cfblk16) -> cfblk20/1
  cfblk20/1 -> cfblk18/1(cfblk1)
  cfblk10/3(cfblk17) -> cfblk21/1
  cfblk21/1 -> cfblk18/3(cfblk12)
  cfblk12/1(cfblk2) -> cfblk22/1
  cfblk22/1 -> cfblk4/1

== system Sample594/cfblk11/cfblk14/cfblk11 ==
  cfblk1 : Inport
  cfblk3 : Bias  Bias=[617680043.966042]
  cfblk4 : Signum
  cfblk5 : PermuteDimensions
  cfblk6 : Subsystem
  cfblk7 : Subsystem
  cfblk8 : Delay
  cfblk2 : Outport
  wires:
  cfblk1/1 -> cfblk5/1, cfblk7/4(cfblk11)
  cfblk3/1 -> cfblk6/1(cfblk1), cfblk7/5(cfblk12)
  cfblk6/2(cfblk10) -> cfblk4/1
  cfblk5/1 -> cfblk7/1(cfblk1), cfblk7/3(cfblk10)
  cfblk7/1(cfblk2) -> cfblk2/1
  cfblk4/1 -> cfblk7/2(cfblk9)
  cfblk6/1(cfblk2) -> cfblk8/1
  cfblk8/1 -> cfblk3/1

== system Sample594/cfblk11/cfblk14/cfblk12 ==
  cfblk1 : Inport
  cfblk10 : Constant  Value=[211579094.084377]  SampleTime=1
  cfblk11 : Subsystem
  cfblk12 : Subsystem
  cfblk13 : Subsystem
  cfblk14 : If  IfExpression=u1 >= 0  SampleTime=1
  cfblk18 : Subsystem  TreatAsAtomicUnit=on
  cfblk19 : Subsystem  TreatAsAtomicUnit=on
  cfblk{20..23} (4 alike) : Delay
  cfblk3 : Delay  DelayLengthSource=Input port
      settings: InputPortMap=u0,p1
  cfblk4 : MinMax  Inputs=3
  cfblk5 : UnaryMinus
  cfblk6 : Math  Operator=log  SaturateOnIntegerOverflow=on
  cfblk7 : UnaryMinus
  cfblk8 : Rounding
  cfblk9 : Product  Inputs=*
  cfblk2 : Outport
  cfblk15 : Outport  Port=2
  cfblk16 : Outport  Port=3
  cfblk17 : Outport  Port=4
  wires:
  cfblk18/1(cfblk2) -> cfblk7/1, cfblk5/1
  cfblk6/1 -> cfblk8/1
  cfblk5/1 -> cfblk16/1, cfblk12/1(cfblk1)
  cfblk1/1 -> cfblk14/1
  cfblk8/1 -> cfblk15/1
  cfblk7/1 -> cfblk9/1
  cfblk12/1(cfblk2) -> cfblk13/1(cfblk1)
  cfblk3/1 -> cfblk12/2(cfblk12), cfblk20/1
  cfblk11/1(cfblk2) -> cfblk19/2(cfblk17), cfblk4/2, cfblk4/3
  cfblk9/1 -> cfblk3/1, cfblk6/1
  cfblk10/1 -> cfblk11/1(cfblk1)
  cfblk19/1(cfblk2) -> cfblk17/1
  cfblk12/3(cfblk14) -> cfblk13/2(cfblk9)
  cfblk12/4(cfblk15) -> cfblk2/1
  cfblk12/5(cfblk16) -> cfblk4/1
  cfblk14/1 -> cfblk18/Action
  cfblk14/2 -> cfblk19/Action
  cfblk20/1 -> cfblk18/2(cfblk10)
  cfblk13/1(cfblk2) -> cfblk21/1
  cfblk21/1 -> cfblk3/2
  cfblk12/2(cfblk13) -> cfblk22/1
  cfblk22/1 -> cfblk19/1(cfblk1)
  cfblk4/1 -> cfblk23/1
  cfblk23/1 -> cfblk18/1(cfblk1)

== system Sample594/cfblk11/cfblk15/cfblk7 ==
  cfblk1 : Inport
  cfblk8 : Inport  Port=2
  cfblk3 : DiscreteTransferFcn
  cfblk4 : DiscreteFir
  cfblk5 : Product
  cfblk6 : Sqrt  Operator=rSqrt  AlgorithmType=Newton-Raphson  SaturateOnIntegerOverflow=on
  cfblk7 : Subsystem
  cfblk9 : Delay
  cfblk2 : Outport
  wires:
  cfblk5/1 -> cfblk6/1
  cfblk4/1 -> cfblk7/1(cfblk1), cfblk7/3(cfblk10)
  cfblk1/1 -> cfblk5/2
  cfblk8/1 -> cfblk4/1
  cfblk7/2(cfblk11) -> cfblk2/1
  cfblk6/1 -> cfblk3/1
  cfblk3/1 -> cfblk7/2(cfblk9)
  cfblk7/1(cfblk2) -> cfblk9/1
  cfblk9/1 -> cfblk5/1

== system Sample594/cfblk11/cfblk15/cfblk8 ==
  cfblk1 : Inport
  cfblk11 : Inport  Port=2
  cfblk12 : Inport  Port=3
  cfblk10 : If  IfExpression=u1 >= 0  SampleTime=1
  cfblk13 : Subsystem  TreatAsAtomicUnit=on
  cfblk14 : Subsystem  TreatAsAtomicUnit=on
  cfblk15 : Delay
  cfblk16 : Delay
  cfblk17 : Delay
  cfblk3 : UnitDelay  SampleTime=-1  HasFrameUpgradeWarning=on
  cfblk4 : Math  Operator=hypot  SaturateOnIntegerOverflow=on
  cfblk5 : Sum  Inputs=|++
  cfblk6 : Constant  Value=[643059211.370470]  SampleTime=1
  cfblk7 : Subsystem
  cfblk8 : Subsystem
  cfblk9 : Subsystem
  cfblk2 : Outport
  wires:
  cfblk14/1(cfblk2) -> cfblk13/1(cfblk1)
  cfblk12/1 -> cfblk3/1
  cfblk6/1 -> cfblk14/1(cfblk1), cfblk7/3(cfblk9)
  cfblk5/1 -> cfblk4/1
  cfblk3/1 -> cfblk4/2
  cfblk9/2(cfblk9) -> cfblk2/1
  cfblk7/1(cfblk2) -> cfblk9/1(cfblk1)
  cfblk11/1 -> cfblk14/2(cfblk13), cfblk8/3(cfblk8)
  cfblk1/1 -> cfblk14/3(cfblk14), cfblk7/1(cfblk1), cfblk7/4(cfblk10)
  cfblk13/1(cfblk2) -> cfblk8/1(cfblk1)
  cfblk14/2(cfblk16) -> cfblk8/2(cfblk7), cfblk7/5(cfblk11)
  cfblk8/1(cfblk2) -> cfblk5/1
  cfblk8/2(cfblk9) -> cfblk5/2, cfblk7/2(cfblk8), cfblk7/6(cfblk12)
  cfblk10/1 -> cfblk13/Action
  cfblk10/2 -> cfblk14/Action
  cfblk4/1 -> cfblk15/1
  cfblk15/1 -> cfblk13/2(cfblk9)
  cfblk9/1(cfblk2) -> cfblk16/1
  cfblk16/1 -> cfblk10/1
  cfblk13/2(cfblk10) -> cfblk17/1
  cfblk17/1 -> cfblk14/4(cfblk15)

== system Sample594/cfblk11/cfblk18/cfblk10 ==
  cfblk1 : Inport
  cfblk13 : Inport  Port=2
  cfblk10 : Subsystem
  cfblk11 : Subsystem
  cfblk12 : Subsystem
  cfblk14 : Delay
  cfblk15 : Delay
  cfblk16 : Delay
  cfblk3 : DiscreteTransferFcn
  cfblk4 : simulink/Discrete/Transfer Fcn Lead or Lag  PoleZ=0.95  ZeroZ=0.75  ICPrevOutput=0.0  ICPrevInput=0.0  DoSatur=off
      settings: SourceProductBaseCode=SL
  cfblk5 : simulink/Math Operations/Slider Gain  gain=1  low=0  high=2
  cfblk6 : Constant  Value=[-636183352.621354]  SampleTime=1
  cfblk7 : Constant  Value=[-539112678.406279]  SampleTime=1
  cfblk8 : Subsystem
  cfblk9 : Subsystem
  cfblk2 : Outport
  wires:
  cfblk6/1 -> cfblk10/1(cfblk1), cfblk8/4(cfblk10)
  cfblk1/1 -> cfblk12/1(cfblk1)
  cfblk13/1 -> cfblk8/1(cfblk1), cfblk9/4(cfblk14)
  cfblk4/1 -> cfblk2/1, cfblk8/3(cfblk9)
  cfblk9/1(cfblk2) -> cfblk4/1
  cfblk9/2(cfblk15) -> cfblk10/2(cfblk11)
  cfblk7/1 -> cfblk12/2(cfblk12), cfblk3/1, cfblk9/3(cfblk13)
  cfblk3/1 -> cfblk5/1, cfblk11/3(cfblk9)
  cfblk10/1(cfblk2) -> cfblk11/1(cfblk1)
  cfblk11/2(cfblk12) -> cfblk8/2(cfblk8)
  cfblk5/1 -> cfblk9/1(cfblk1)
  cfblk8/1(cfblk2) -> cfblk15/1, cfblk16/1
  cfblk12/1(cfblk2) -> cfblk10/3(cfblk12)
  cfblk12/2(cfblk15) -> cfblk9/2(cfblk12)
  cfblk12/3(cfblk16) -> cfblk11/2(cfblk8), cfblk11/5(cfblk11)
  cfblk11/1(cfblk2) -> cfblk14/1
  cfblk14/1 -> cfblk12/3(cfblk13)
  cfblk15/1 -> cfblk12/4(cfblk14)
  cfblk16/1 -> cfblk11/4(cfblk10)

== system Sample594/cfblk11/cfblk18/cfblk11 ==
  cfblk1 : Inport
  cfblk12 : Inport  Port=2
  cfblk13 : Inport  Port=3
  cfblk10 : Subsystem
  cfblk11 : Subsystem
  cfblk14 : Delay
  cfblk15 : Delay
  cfblk16 : Delay
  cfblk3 : Delay  ShowEnablePort=on
      settings: InputPortMap=u0,e6
  cfblk4 : simulink/Math Operations/MinMax Running Resettable  Function=min  vinit=0.0
  cfblk5 : Sum
  cfblk6 : Sum  Inputs=|++
  cfblk7 : Constant  Value=[-143653998.695095]  SampleTime=1
  cfblk8 : Subsystem
  cfblk9 : Subsystem
  cfblk2 : Outport
  wires:
  cfblk10/1(cfblk2) -> cfblk8/1(cfblk1)
  cfblk7/1 -> cfblk11/1(cfblk1), cfblk9/3(cfblk10)
  cfblk5/1 -> cfblk11/2(cfblk16)
  cfblk3/1 -> cfblk10/1(cfblk1)
  cfblk9/1(cfblk2) -> cfblk4/2, cfblk16/1
  cfblk1/1 -> cfblk2/1, cfblk3/2
  cfblk13/1 -> cfblk3/1, cfblk6/2, cfblk9/4(cfblk11)
  cfblk11/2(cfblk17) -> cfblk4/1
  cfblk12/1 -> cfblk6/1, cfblk9/2(cfblk9), cfblk8/3(cfblk7)
  cfblk6/1 -> cfblk9/1(cfblk1)
  cfblk8/1(cfblk2) -> cfblk5/2, cfblk9/5(cfblk12)
  cfblk11/1(cfblk2) -> cfblk14/1
  cfblk14/1 -> cfblk5/1
  cfblk4/1 -> cfblk15/1
  cfblk15/1 -> cfblk10/2(cfblk10)
  cfblk16/1 -> cfblk8/2(cfblk6)

== system Sample594/cfblk11/cfblk18/cfblk9 ==
  cfblk1 : Inport
  cfblk12 : Inport  Port=2
  cfblk13 : Inport  Port=3
  cfblk14 : Inport  Port=4
  cfblk10 : Subsystem
  cfblk11 : Subsystem
  cfblk15 : Delay
  cfblk3 : Delay
  cfblk4 : DiscreteStateSpace  SampleTime=-1
  cfblk5 : Polyval  Coefs=[ +2.081618890e-019, -1.441693666e-014, +4.719686976e-010, -8.536869453e-006, +1.621573104e-001, -8.087801117e+001 ]
  cfblk6 : Product  Inputs=**
  cfblk7 : MinMax  Inputs=2
  cfblk8 : Constant  Value=[-689609996.566453]  SampleTime=1
  cfblk9 : Constant  Value=[-386197627.716200]  SampleTime=1
  cfblk2 : Outport
  wires:
  cfblk13/1 -> cfblk11/1(cfblk1)
  cfblk11/1(cfblk2) -> cfblk3/1
  cfblk1/1 -> cfblk10/2(cfblk9)
  cfblk7/1 -> cfblk4/1
  cfblk10/1(cfblk2) -> cfblk6/1
  cfblk14/1 -> cfblk2/1
  cfblk8/1 -> cfblk5/1
  cfblk4/1 -> cfblk6/2
  cfblk9/1 -> cfblk7/1
  cfblk3/1 -> cfblk7/2
  cfblk6/1 -> cfblk15/1
  cfblk15/1 -> cfblk10/1(cfblk1)

== system Sample594/cfblk11/cfblk19/cfblk6 ==
  cfblk1 : Inport
  cfblk11 : Inport  Port=2
  cfblk10 : Subsystem
  cfblk15 : Delay
  cfblk16 : Delay
  cfblk3 : Sum  Inputs=+
  cfblk4 : Math  Operator=rem  SaturateOnIntegerOverflow=on
  cfblk5 : Gain  Gain=[-93419522.347786]
  cfblk6 : Assignment  DiagnosticForDimensions=Warning  IndexOptions=Index vector (dialog)  Indices=1  OutputSizes=1
  cfblk7 : DotProduct  InputSameDT=on  OutDataTypeStr=Inherit: Inherit via internal rule
  cfblk8 : Subsystem
  cfblk9 : Subsystem
  cfblk2 : Outport
  cfblk12 : Outport  Port=2
  cfblk13 : Outport  Port=3
  cfblk14 : Outport  Port=4
  wires:
  cfblk7/1 -> cfblk8/1(cfblk1), cfblk6/2
  cfblk1/1 -> cfblk14/1, cfblk9/2(cfblk10)
  cfblk11/1 -> cfblk8/2(cfblk8), cfblk9/1(cfblk1)
  cfblk3/1 -> cfblk12/1
  cfblk10/2(cfblk17) -> cfblk3/1, cfblk13/1
  cfblk8/1(cfblk2) -> cfblk2/1
  cfblk9/1(cfblk2) -> cfblk7/2, cfblk6/1
  cfblk8/2(cfblk10) -> cfblk5/1
  cfblk4/1 -> cfblk10/1(cfblk1), cfblk10/3(cfblk16)
  cfblk6/1 -> cfblk10/2(cfblk15), cfblk8/3(cfblk9)
  cfblk8/3(cfblk11) -> cfblk4/2
  cfblk5/1 -> cfblk15/1
  cfblk15/1 -> cfblk7/1
  cfblk10/1(cfblk2) -> cfblk16/1
  cfblk16/1 -> cfblk4/1

== system Sample594/cfblk11/cfblk19/cfblk7 ==
  cfblk1 : Inport
  cfblk3 : Constant  Value=[718631614.067329]  SampleTime=1
  cfblk4 : Constant  Value=[-970143308.981806]  SampleTime=1
  cfblk5 : Subsystem
  cfblk6 : Subsystem
  cfblk7 : Subsystem
  cfblk8 : Subsystem
  cfblk2 : Outport
  wires:
  cfblk5/1(cfblk2) -> cfblk6/1(cfblk1)
  cfblk7/1(cfblk2) -> cfblk2/1
  cfblk3/1 -> cfblk7/1(cfblk1)
  cfblk7/2(cfblk13) -> cfblk8/1(cfblk1)
  cfblk6/1(cfblk2) -> cfblk8/2(cfblk9)
  cfblk7/3(cfblk14) -> cfblk5/1(cfblk1)
  cfblk4/1 -> cfblk5/2(cfblk7)

== system Sample594/cfblk12/cfblk10/cfblk10 ==
  cfblk1 : Inport
  cfblk10 : Inport  Port=2
  cfblk11 : Inport  Port=3
  cfblk12 : Delay
  cfblk3 : simulink/Discrete/Tapped Delay  vinit=0.0  samptime=-1  NumDelays=1  DelayOrder=Oldest  includeCurrent=off
  cfblk4 : simulink/Discrete/Transfer Fcn Lead or Lag  PoleZ=0.95  ZeroZ=0.75  ICPrevOutput=0.0  ICPrevInput=0.0  DoSatur=off
      settings: SourceProductBaseCode=SL
  cfblk5 : Assignment  DiagnosticForDimensions=Warning  IndexOptions=Index vector (dialog)  Indices=1  OutputSizes=1
  cfblk6 : Constant  Value=[616464398.117188]  SampleTime=1
  cfblk7 : Constant  Value=[-723924681.229688]  SampleTime=1
  cfblk8 : Subsystem
  cfblk9 : Subsystem
  cfblk2 : Outport
  wires:
  cfblk6/1 -> cfblk8/1(cfblk1)
  cfblk1/1 -> cfblk4/1
  cfblk8/1(cfblk2) -> cfblk3/1
  cfblk10/1 -> cfblk5/1
  cfblk7/1 -> cfblk2/1
  cfblk11/1 -> cfblk5/2
  cfblk4/1 -> cfblk8/3(cfblk7)
  cfblk3/1 -> cfblk9/1(cfblk1)
  cfblk5/1 -> cfblk8/4(cfblk8)
  cfblk9/1(cfblk2) -> cfblk12/1
  cfblk12/1 -> cfblk8/2(cfblk6)

== system Sample594/cfblk12/cfblk10/cfblk9 ==
  cfblk1 : Inport
  cfblk10 : Inport  Port=2
  cfblk11 : Delay
  cfblk12 : Delay
  cfblk3 : DiscreteZeroPole  Poles=[0 0.5]  Gain=1  SampleTime=-1
  cfblk4 : simulink/Math Operations/MinMax Running Resettable  Function=min  vinit=0.0
  cfblk5 : Sum  Inputs=+-
  cfblk6 : Gain  Gain=[-609634712.328249]
  cfblk7 : Assignment  DiagnosticForDimensions=Warning  IndexOptions=Index vector (dialog)  Indices=1  OutputSizes=1
  cfblk8 : Constant  Value=[-166273062.301539]  SampleTime=1
  cfblk9 : Subsystem
  cfblk2 : Outport
  wires:
  cfblk1/1 -> cfblk5/1
  cfblk4/1 -> cfblk6/1
  cfblk6/1 -> cfblk9/1(cfblk1), cfblk12/1
  cfblk8/1 -> cfblk2/1
  cfblk3/1 -> cfblk4/2
  cfblk10/1 -> cfblk7/1
  cfblk9/1(cfblk2) -> cfblk7/2
  cfblk5/1 -> cfblk3/1
  cfblk7/1 -> cfblk11/1
  cfblk11/1 -> cfblk4/1
  cfblk12/1 -> cfblk5/2

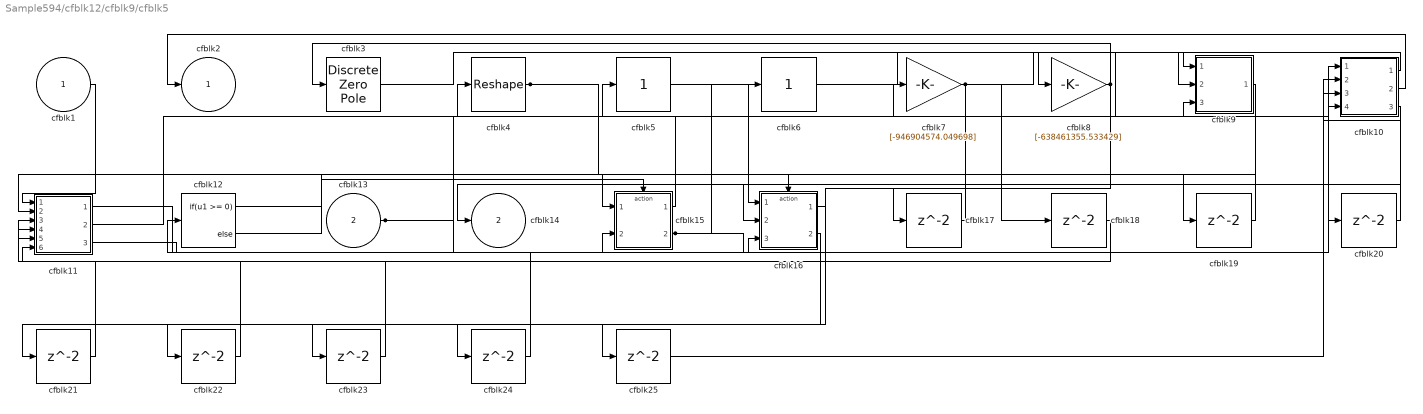
== system Sample594/cfblk12/cfblk9/cfblk5 ==
  cfblk1 : Inport
  cfblk13 : Inport  Port=2
  cfblk10 : Subsystem
  cfblk11 : Subsystem
  cfblk12 : If  IfExpression=u1 >= 0  SampleTime=1
  cfblk15 : Subsystem  TreatAsAtomicUnit=on
  cfblk16 : Subsystem  TreatAsAtomicUnit=on
  cfblk{17..25} (9 alike) : Delay
  cfblk3 : DiscreteZeroPole  Poles=[0 0.5]  Gain=1  SampleTime=-1
  cfblk4 : Reshape
  cfblk5 : simulink/Math Operations/Slider Gain  gain=1  low=0  high=2
  cfblk6 : simulink/Math Operations/Slider Gain  gain=1  low=0  high=2
  cfblk7 : Gain  Gain=[-946904574.049698]
  cfblk8 : Gain  Gain=[-638461355.533429]
  cfblk9 : Subsystem
  cfblk2 : Outport
  cfblk14 : Outport  Port=2
  wires:
  cfblk9/1(cfblk2) -> cfblk14/1
  cfblk15/1(cfblk2) -> cfblk4/1
  cfblk4/1 -> cfblk9/3(cfblk15), cfblk19/1
  cfblk6/1 -> cfblk8/1
  cfblk8/1 -> cfblk3/1, cfblk21/1, cfblk22/1, cfblk23/1
  cfblk10/1(cfblk2) -> cfblk7/1
  cfblk1/1 -> cfblk11/1(cfblk1)
  cfblk7/1 -> cfblk9/1(cfblk1), cfblk17/1, cfblk18/1
  cfblk5/1 -> cfblk16/1(cfblk1)
  cfblk11/1(cfblk2) -> cfblk10/1(cfblk1)
  cfblk10/2(cfblk15) -> cfblk2/1
  cfblk3/1 -> cfblk9/2(cfblk14)
  cfblk15/2(cfblk12) -> cfblk6/1, cfblk20/1
  cfblk13/1 -> cfblk10/4(cfblk14), cfblk15/2(cfblk11)
  cfblk10/3(cfblk16) -> cfblk16/2(cfblk14)
  cfblk11/2(cfblk15) -> cfblk5/1
  cfblk11/3(cfblk16) -> cfblk16/3(cfblk15)
  cfblk12/1 -> cfblk15/Action
  cfblk12/2 -> cfblk16/Action
  cfblk17/1 -> cfblk11/2(cfblk10)
  cfblk18/1 -> cfblk11/3(cfblk11)
  cfblk19/1 -> cfblk15/1(cfblk1)
  cfblk20/1 -> cfblk10/3(cfblk13)
  cfblk21/1 -> cfblk11/4(cfblk12)
  cfblk22/1 -> cfblk11/5(cfblk13)
  cfblk23/1 -> cfblk11/6(cfblk14)
  cfblk16/1(cfblk2) -> cfblk24/1
  cfblk24/1 -> cfblk12/1
  cfblk16/2(cfblk16) -> cfblk25/1
  cfblk25/1 -> cfblk10/2(cfblk12)

== system Sample594/cfblk12/cfblk9/cfblk6 ==
  cfblk1 : Inport
  cfblk9 : Inport  Port=2
  cfblk10 : Delay
  cfblk11 : Delay
  cfblk3 : DiscreteFir
  cfblk4 : Product  Inputs=**
  cfblk5 : simulink/Math Operations/Slider Gain  gain=1  low=0  high=2
  cfblk6 : Subsystem
  cfblk7 : Subsystem
  cfblk8 : Subsystem
  cfblk2 : Outport
  wires:
  cfblk5/1 -> cfblk6/1(cfblk1), cfblk7/4(cfblk9), cfblk4/1, cfblk4/2
  cfblk7/1(cfblk2) -> cfblk3/1
  cfblk1/1 -> cfblk8/1(cfblk1)
  cfblk4/1 -> cfblk8/2(cfblk16), cfblk2/1
  cfblk9/1 -> cfblk5/1
  cfblk6/1(cfblk2) -> cfblk10/1, cfblk11/1
  cfblk8/1(cfblk2) -> cfblk7/2(cfblk7)
  cfblk8/2(cfblk17) -> cfblk7/3(cfblk8)
  cfblk3/1 -> cfblk6/2(cfblk7)
  cfblk10/1 -> cfblk7/1(cfblk1)
  cfblk11/1 -> cfblk7/5(cfblk10)

== system Sample594/cfblk12/cfblk9/cfblk7 ==
  cfblk1 : Inport
  cfblk{10..13} (4 alike) : Delay
  cfblk3 : simulink/Discrete/Transfer Fcn First Order  PoleZ=0.95  ICPrevOutput=0.0  DoSatur=off
  cfblk4 : DiscreteIntegrator  SampleTime=-1  ICPrevOutput=DiscIntNeverNeededParam  ICPrevScaledInput=DiscIntNeverNeededParam
  cfblk5 : DiscreteFilter
  cfblk6 : Polyval  Coefs=[ +2.081618890e-019, -1.441693666e-014, +4.719686976e-010, -8.536869453e-006, +1.621573104e-001, -8.087801117e+001 ]
  cfblk7 : Subsystem
  cfblk8 : Subsystem
  cfblk9 : Subsystem
  cfblk2 : Outport
  wires:
  cfblk6/1 -> cfblk7/4(cfblk9), cfblk13/1
  cfblk1/1 -> cfblk4/1
  cfblk4/1 -> cfblk9/2(cfblk12), cfblk8/3(cfblk12)
  cfblk5/1 -> cfblk6/1
  cfblk7/1(cfblk2) -> cfblk2/1
  cfblk9/1(cfblk2) -> cfblk7/1(cfblk1)
  cfblk9/2(cfblk14) -> cfblk5/1
  cfblk7/2(cfblk10) -> cfblk3/1
  cfblk3/1 -> cfblk8/1(cfblk1), cfblk8/2(cfblk11), cfblk8/4(cfblk13)
  cfblk8/2(cfblk14) -> cfblk11/1, cfblk12/1
  cfblk8/1(cfblk2) -> cfblk10/1
  cfblk10/1 -> cfblk7/2(cfblk7)
  cfblk11/1 -> cfblk7/3(cfblk8)
  cfblk12/1 -> cfblk9/3(cfblk13)
  cfblk13/1 -> cfblk9/1(cfblk1)

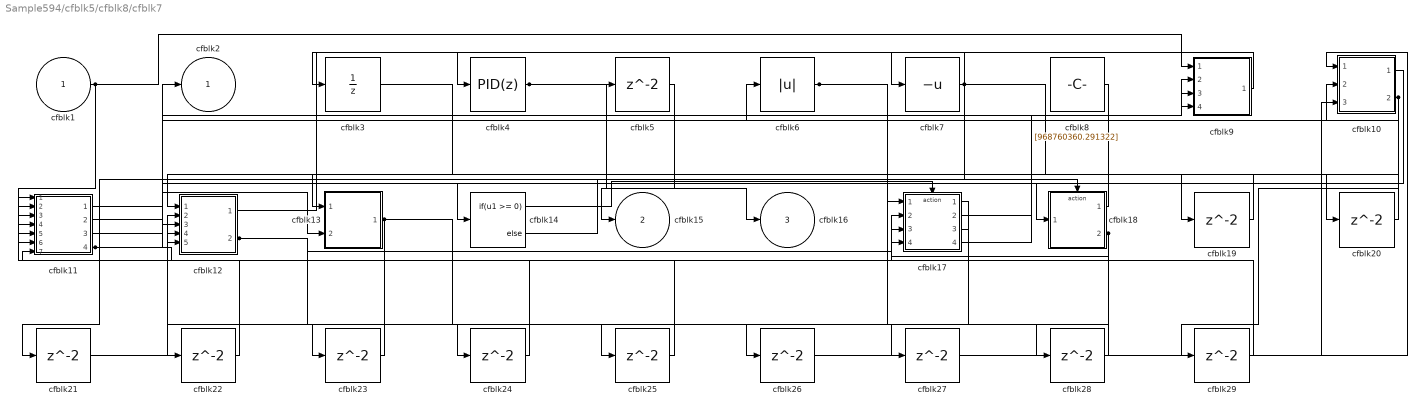
== system Sample594/cfblk5/cfblk8/cfblk7 ==
  cfblk1 : Inport
  cfblk10 : Subsystem
  cfblk11 : Subsystem
  cfblk12 : Subsystem
  cfblk13 : Subsystem
  cfblk14 : If  IfExpression=u1 >= 0  SampleTime=1
  cfblk17 : Subsystem  TreatAsAtomicUnit=on
  cfblk18 : Subsystem  TreatAsAtomicUnit=on
  cfblk{5,19..29} (12 alike) : Delay  SampleTime=1
  cfblk3 : UnitDelay  HasFrameUpgradeWarning=on
  cfblk4 : pid_lib/PID Controller  Controller=PID  Form=Parallel  TimeDomain=Discrete-time  UseExternalTs=off  SampleTime=1  IntegratorMethod=Forward Euler  FilterMethod=Forward Euler  ControllerParametersSource=internal  P=1  I=1  D=0  UseFilter=on  N=100  TunerSelectOption=Transfer Function Based (PID Tuner App)  InitialConditionSource=internal  InitialConditionForIntegrator=0  InitialConditionForFilter=0  DifferentiatorICPrevScaledInput=0  ExternalReset=none  TrackingMode=off  Kt=1  LimitOutput=off  SatLimitsSource=internal  UpperSaturationLimit=inf  LowerSaturationLimit=-inf  LinearizeAsGain=off  AntiWindupMode=none  Kb=1  POutMin=[]  POutMax=[]  IOutMin=[]  IOutMax=[]  DOutMin=[]  DOutMax=[]  NOutMin=[]  NOutMax=[]  SumOutMin=[]  SumOutMax=[]  SaturationOutMin=[]  SaturationOutMax=[]  PParamMin=[]  PParamMax=[]  IParamMin=[]  IParamMax=[]  DParamMin=[]  DParamMax=[]  NParamMin=[]  NParamMax=[]  KbParamMin=[]  KbParamMax=[]  KtParamMin=[]  KtParamMax=[]  KbOutMin=[]  KbOutMax=[]  KtOutMin=[]  KtOutMax=[]  IntegratorOutMin=[]  IntegratorOutMax=[]  FilterOutMin=[]  FilterOutMax=[]  SumI1OutMin=[]  SumI1OutMax=[]  SumI2OutMin=[]  SumI2OutMax=[]  SumI3OutMin=[]  SumI3OutMax=[]  SumI4OutMin=[]  SumI4OutMax=[]  SumDOutMin=[]  SumDOutMax=[]  DifferentiatorOutMin=[]  DifferentiatorOutMax=[]  FilterDiffOutCoefMin=[]  FilterDiffOutCoefMax=[]  ReciprocalOutMin=[]  ReciprocalOutMax=[]  SumDenOutMin=[]  SumDenOutMax=[]  SumNumOutMin=[]  SumNumOutMax=[]  DivideOutMin=[]  DivideOutMax=[]  UdiffTsProdOutMin=[]  UdiffTsProdOutMax=[]  NTsProdOutMin=[]  NTsProdOutMax=[]  UintegralTsProdOutMin=[]  UintegralTsProdOutMax=[]  UngainTsProdOutMin=[]  UngainTsProdOutMax=[]  IntegratorContinuousStateAttributes=''  IntegratorStateMustResolveToSignalObject=off  IntegratorRTWStateStorageClass=Auto  FilterContinuousStateAttributes=''  FilterStateMustResolveToSignalObject=off  FilterRTWStateStorageClass=Auto  ParallelPVariant=InternalParameters  IdealPVariant=Disabled  IVariant=InternalParameters  DVariant=InternalParameters  IntegratorVariant=Discrete  SatVariant=Disabled  AWVariant=Passthrough  PCopyVariant=Disabled  TRVariant=Disabled  FdbkBlocksVariant=Forward  IdealPFdbkVariant=Disabled  SatFdbkVariant=Disabled  DerivativeFilterVariant=ForwardEulerFilter  NVariant=InternalParameters  NCopyVariant=Disabled  FilterICVariant=InternalICsFilter  IntegratorICVariant=InternalICs  ExternalResetVariant=Disabled  TRSumVariant=Passthrough  SumFdbkVariant=Disabled  SumVariant=Sum_PID  TsampFilterVariant=InternalTs  TsampNgainVariant=Passthrough  TsampIntegralVariant=Passthrough  ExternalSaturationOutDataTypeStr=Inherit: Same as second input
  cfblk6 : Abs
  cfblk7 : UnaryMinus
  cfblk8 : Constant  Value=[968760360.291322]  SampleTime=1
  cfblk9 : Subsystem
  cfblk2 : Outport
  cfblk15 : Outport  Port=2
  cfblk16 : Outport  Port=3
  wires:
  cfblk4/1 -> cfblk16/1, cfblk5/1
  cfblk12/1(cfblk2) -> cfblk7/1
  cfblk10/1(cfblk2) -> cfblk18/1(cfblk1)
  cfblk7/1 -> cfblk3/1, cfblk19/1, cfblk21/1
  cfblk13/1(cfblk2) -> cfblk12/2(cfblk7), cfblk12/4(cfblk9), cfblk25/1
  cfblk1/1 -> cfblk9/1(cfblk1), cfblk11/4(cfblk10)
  cfblk9/1(cfblk2) -> cfblk4/1
  cfblk18/1(cfblk2) -> cfblk12/3(cfblk8)
  cfblk11/1(cfblk2) -> cfblk13/2(cfblk14)
  cfblk17/2(cfblk13) -> cfblk9/2(cfblk15)
  cfblk10/2(cfblk7) -> cfblk6/1, cfblk29/1
  cfblk6/1 -> cfblk17/1(cfblk1), cfblk28/1
  cfblk8/1 -> cfblk14/1
  cfblk12/2(cfblk11) -> cfblk17/2(cfblk10), cfblk24/1
  cfblk11/2(cfblk14) -> cfblk2/1
  cfblk18/2(cfblk7) -> cfblk17/4(cfblk12), cfblk26/1, cfblk27/1
  cfblk17/4(cfblk15) -> cfblk9/3(cfblk16)
  cfblk5/1 -> cfblk15/1
  cfblk11/3(cfblk15) -> cfblk10/2(cfblk5)
  cfblk11/4(cfblk16) -> cfblk17/3(cfblk11), cfblk9/4(cfblk17)
  cfblk14/1 -> cfblk17/Action
  cfblk14/2 -> cfblk18/Action
  cfblk19/1 -> cfblk12/1(cfblk1)
  cfblk3/1 -> cfblk20/1
  cfblk20/1 -> cfblk13/1(cfblk1)
  cfblk21/1 -> cfblk12/5(cfblk10)
  cfblk17/1(cfblk2) -> cfblk22/1
  cfblk22/1 -> cfblk11/1(cfblk1)
  cfblk17/3(cfblk14) -> cfblk23/1
  cfblk23/1 -> cfblk11/2(cfblk8)
  cfblk24/1 -> cfblk11/6(cfblk12)
  cfblk25/1 -> cfblk11/3(cfblk9)
  cfblk26/1 -> cfblk10/1(cfblk1)
  cfblk27/1 -> cfblk10/3(cfblk6)
  cfblk28/1 -> cfblk11/7(cfblk13)
  cfblk29/1 -> cfblk11/5(cfblk11)
